simulink model "Lv_topo4"  (R2024a)
settings: Solver=ode4  StartTime=0.0  StopTime=1  FixedStep=5e-05  RelTol=1e-3
libraries: spsSeriesRLCBranchLib x38, spsThreePhaseSeriesRLCBranchLib x18, spsCurrentMeasurementLib x16, spsPowerLib x16, spsSeriesRLCLoadLib x16, spsVoltageMeasurementLib x16, spsThreePhaseVIMeasurementLib x2, spsGroundLib x2, spsPower3phInstantaneousLib x2, spsThreePhaseTransformerTwoWindingsLib x2, spsThreePhaseSourceLib x1, sps_lib x1
(part 2 of 2)

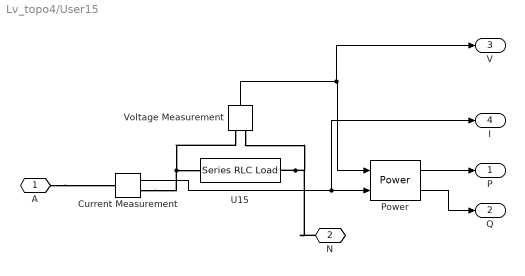
== system Lv_topo4/User15 ==
  Current Measurement : spsCurrentMeasurementLib/Current Measurement  PhasorSimulation=off  OutputType=Complex  PSBequivalent=0
  Power : spsPowerLib/Power  Freq=50  Vinit=[1, 0]  Iinit=[1, 0]  Ts=0
  U15 : spsSeriesRLCLoadLib/Series RLC Load  LConnTagsString=a  RConnTagsString=__new0  NominalVoltage=220  NominalFrequency=50  ActivePower=1045  InductivePower=503.5  CapacitivePower=0  Setx0=off  InitialVoltage=0  SetiL0=off  InitialCurrent=0  Measurements=None  LoadType=constant PQ
  Voltage Measurement : spsVoltageMeasurementLib/Voltage Measurement  PhasorSimulation=off  OutputType=Complex  PSBequivalent=0
  A : PMIOPort  Side=Left
  N : PMIOPort  Port=2  Side=Right
  P : Outport
  Q : Outport  Port=2
  V : Outport  Port=3
  I : Outport  Port=4
  wires:
  Power/1 -> P/1
  Power/2 -> Q/1
  Voltage Measurement/1 -> V/1, Power/1
  Current Measurement/1 -> I/1, Power/2
  connections:
  U15/RConn1 -- Voltage Measurement/LConn2 -- N/RConn1
  Current Measurement/RConn1 -- Voltage Measurement/LConn1 -- U15/LConn1
  A/RConn1 -- Current Measurement/LConn1

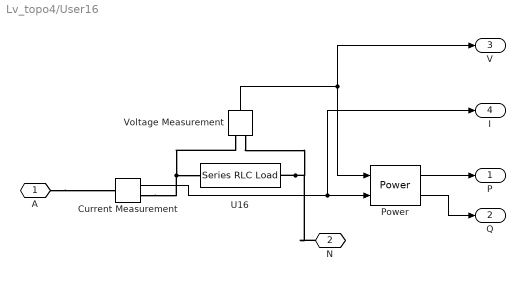
== system Lv_topo4/User16 ==
  Current Measurement : spsCurrentMeasurementLib/Current Measurement  PhasorSimulation=off  OutputType=Complex  PSBequivalent=0
  Power : spsPowerLib/Power  Freq=50  Vinit=[1, 0]  Iinit=[1, 0]  Ts=0
  U16 : spsSeriesRLCLoadLib/Series RLC Load  LConnTagsString=a  RConnTagsString=__new0  NominalVoltage=220  NominalFrequency=50  ActivePower=847  InductivePower=286  CapacitivePower=0  Setx0=off  InitialVoltage=0  SetiL0=off  InitialCurrent=0  Measurements=None  LoadType=constant PQ
  Voltage Measurement : spsVoltageMeasurementLib/Voltage Measurement  PhasorSimulation=off  OutputType=Complex  PSBequivalent=0
  A : PMIOPort  Side=Left
  N : PMIOPort  Port=2  Side=Right
  P : Outport
  Q : Outport  Port=2
  V : Outport  Port=3
  I : Outport  Port=4
  wires:
  Power/1 -> P/1
  Power/2 -> Q/1
  Current Measurement/1 -> I/1, Power/2
  Voltage Measurement/1 -> V/1, Power/1
  connections:
  U16/RConn1 -- Voltage Measurement/LConn2 -- N/RConn1
  Current Measurement/RConn1 -- Voltage Measurement/LConn1 -- U16/LConn1
  A/RConn1 -- Current Measurement/LConn1

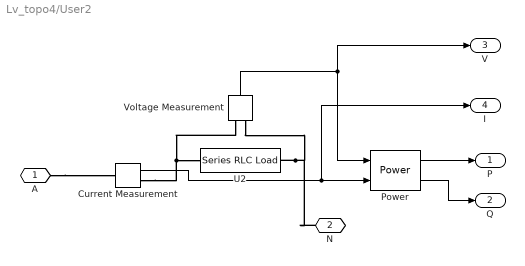
== system Lv_topo4/User2 ==
  Current Measurement : spsCurrentMeasurementLib/Current Measurement  PhasorSimulation=off  OutputType=Complex  PSBequivalent=0
  Power : spsPowerLib/Power  Freq=50  Vinit=[1, 0]  Iinit=[1, 0]  Ts=0
  U2 : spsSeriesRLCLoadLib/Series RLC Load  LConnTagsString=a  RConnTagsString=__new0  NominalVoltage=220  NominalFrequency=50  ActivePower=840  InductivePower=410  CapacitivePower=0  Setx0=off  InitialVoltage=0  SetiL0=off  InitialCurrent=0  Measurements=None  LoadType=constant PQ
  Voltage Measurement : spsVoltageMeasurementLib/Voltage Measurement  PhasorSimulation=off  OutputType=Complex  PSBequivalent=0
  A : PMIOPort  Side=Left
  N : PMIOPort  Port=2  Side=Right
  P : Outport
  Q : Outport  Port=2
  V : Outport  Port=3
  I : Outport  Port=4
  wires:
  Power/1 -> P/1
  Power/2 -> Q/1
  Voltage Measurement/1 -> V/1, Power/1
  Current Measurement/1 -> I/1, Power/2
  connections:
  U2/RConn1 -- Voltage Measurement/LConn2 -- N/RConn1
  Current Measurement/RConn1 -- Voltage Measurement/LConn1 -- U2/LConn1
  A/RConn1 -- Current Measurement/LConn1

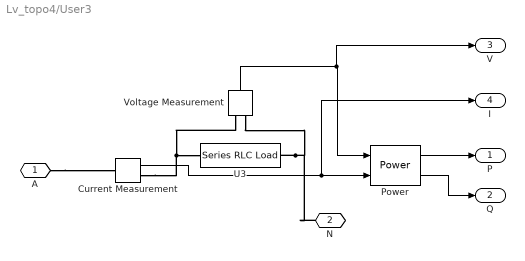
== system Lv_topo4/User3 ==
  Current Measurement : spsCurrentMeasurementLib/Current Measurement  PhasorSimulation=off  OutputType=Complex  PSBequivalent=0
  Power : spsPowerLib/Power  Freq=50  Vinit=[1, 0]  Iinit=[1, 0]  Ts=0
  U3 : spsSeriesRLCLoadLib/Series RLC Load  LConnTagsString=a  RConnTagsString=__new0  NominalVoltage=220  NominalFrequency=50  ActivePower=729.6  InductivePower=355.2  CapacitivePower=0  Setx0=off  InitialVoltage=0  SetiL0=off  InitialCurrent=0  Measurements=None  LoadType=constant PQ
  Voltage Measurement : spsVoltageMeasurementLib/Voltage Measurement  PhasorSimulation=off  OutputType=Complex  PSBequivalent=0
  A : PMIOPort  Side=Left
  N : PMIOPort  Port=2  Side=Right
  P : Outport
  Q : Outport  Port=2
  V : Outport  Port=3
  I : Outport  Port=4
  wires:
  Power/1 -> P/1
  Power/2 -> Q/1
  Current Measurement/1 -> I/1, Power/2
  Voltage Measurement/1 -> V/1, Power/1
  connections:
  U3/RConn1 -- Voltage Measurement/LConn2 -- N/RConn1
  Current Measurement/RConn1 -- Voltage Measurement/LConn1 -- U3/LConn1
  A/RConn1 -- Current Measurement/LConn1

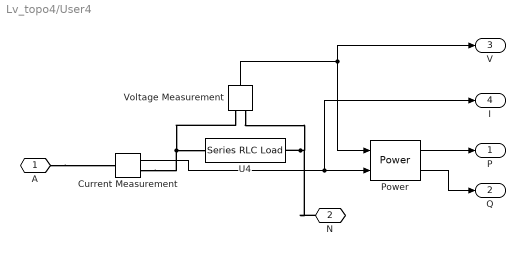
== system Lv_topo4/User4 ==
  Current Measurement : spsCurrentMeasurementLib/Current Measurement  PhasorSimulation=off  OutputType=Complex  PSBequivalent=0
  Power : spsPowerLib/Power  Freq=50  Vinit=[1, 0]  Iinit=[1, 0]  Ts=0
  U4 : spsSeriesRLCLoadLib/Series RLC Load  LConnTagsString=a  RConnTagsString=__new0  NominalVoltage=220  NominalFrequency=50  ActivePower=720  InductivePower=351  CapacitivePower=0  Setx0=off  InitialVoltage=0  SetiL0=off  InitialCurrent=0  Measurements=None  LoadType=constant PQ
  Voltage Measurement : spsVoltageMeasurementLib/Voltage Measurement  PhasorSimulation=off  OutputType=Complex  PSBequivalent=0
  A : PMIOPort  Side=Left
  N : PMIOPort  Port=2  Side=Right
  P : Outport
  Q : Outport  Port=2
  V : Outport  Port=3
  I : Outport  Port=4
  wires:
  Power/1 -> P/1
  Power/2 -> Q/1
  Voltage Measurement/1 -> V/1, Power/1
  Current Measurement/1 -> I/1, Power/2
  connections:
  U4/RConn1 -- Voltage Measurement/LConn2 -- N/RConn1
  Current Measurement/RConn1 -- Voltage Measurement/LConn1 -- U4/LConn1
  A/RConn1 -- Current Measurement/LConn1

== system Lv_topo4/User5 ==
  Current Measurement : spsCurrentMeasurementLib/Current Measurement  PhasorSimulation=off  OutputType=Complex  PSBequivalent=0
  Power : spsPowerLib/Power  Freq=50  Vinit=[1, 0]  Iinit=[1, 0]  Ts=0
  U5 : spsSeriesRLCLoadLib/Series RLC Load  LConnTagsString=a  RConnTagsString=__new0  NominalVoltage=220  NominalFrequency=50  ActivePower=1317.5  InductivePower=641.75  CapacitivePower=0  Setx0=off  InitialVoltage=0  SetiL0=off  InitialCurrent=0  Measurements=None  LoadType=constant PQ
  Voltage Measurement : spsVoltageMeasurementLib/Voltage Measurement  PhasorSimulation=off  OutputType=Complex  PSBequivalent=0
  A : PMIOPort  Side=Left
  N : PMIOPort  Port=2  Side=Right
  P : Outport
  Q : Outport  Port=2
  V : Outport  Port=3
  I : Outport  Port=4
  wires:
  Power/1 -> P/1
  Power/2 -> Q/1
  Current Measurement/1 -> I/1, Power/2
  Voltage Measurement/1 -> V/1, Power/1
  connections:
  U5/RConn1 -- Voltage Measurement/LConn2 -- N/RConn1
  Current Measurement/RConn1 -- Voltage Measurement/LConn1 -- U5/LConn1
  A/RConn1 -- Current Measurement/LConn1

== system Lv_topo4/User6 ==
  Current Measurement : spsCurrentMeasurementLib/Current Measurement  PhasorSimulation=off  OutputType=Complex  PSBequivalent=0
  Power : spsPowerLib/Power  Freq=50  Vinit=[1, 0]  Iinit=[1, 0]  Ts=0
  U6 : spsSeriesRLCLoadLib/Series RLC Load  LConnTagsString=a  RConnTagsString=__new0  NominalVoltage=220  NominalFrequency=50  ActivePower=1071  InductivePower=518.5  CapacitivePower=0  Setx0=off  InitialVoltage=0  SetiL0=off  InitialCurrent=0  Measurements=None  LoadType=constant PQ
  Voltage Measurement : spsVoltageMeasurementLib/Voltage Measurement  PhasorSimulation=off  OutputType=Complex  PSBequivalent=0
  A : PMIOPort  Side=Left
  N : PMIOPort  Port=2  Side=Right
  P : Outport
  Q : Outport  Port=2
  V : Outport  Port=3
  I : Outport  Port=4
  wires:
  Power/1 -> P/1
  Power/2 -> Q/1
  Voltage Measurement/1 -> V/1, Power/1
  Current Measurement/1 -> I/1, Power/2
  connections:
  U6/RConn1 -- Voltage Measurement/LConn2 -- N/RConn1
  Current Measurement/RConn1 -- Voltage Measurement/LConn1 -- U6/LConn1
  A/RConn1 -- Current Measurement/LConn1

== system Lv_topo4/User7 ==
  Current Measurement : spsCurrentMeasurementLib/Current Measurement  PhasorSimulation=off  OutputType=Complex  PSBequivalent=0
  Power : spsPowerLib/Power  Freq=50  Vinit=[1, 0]  Iinit=[1, 0]  Ts=0
  U7 : spsSeriesRLCLoadLib/Series RLC Load  LConnTagsString=a  RConnTagsString=__new0  NominalVoltage=220  NominalFrequency=50  ActivePower=570  InductivePower=275  CapacitivePower=0  Setx0=off  InitialVoltage=0  SetiL0=off  InitialCurrent=0  Measurements=None  LoadType=constant PQ
  Voltage Measurement : spsVoltageMeasurementLib/Voltage Measurement  PhasorSimulation=off  OutputType=Complex  PSBequivalent=0
  A : PMIOPort  Side=Left
  N : PMIOPort  Port=2  Side=Right
  P : Outport
  Q : Outport  Port=2
  V : Outport  Port=3
  I : Outport  Port=4
  wires:
  Power/1 -> P/1
  Power/2 -> Q/1
  Current Measurement/1 -> I/1, Power/2
  Voltage Measurement/1 -> V/1, Power/1
  connections:
  U7/RConn1 -- Voltage Measurement/LConn2 -- N/RConn1
  Current Measurement/RConn1 -- Voltage Measurement/LConn1 -- U7/LConn1
  A/RConn1 -- Current Measurement/LConn1

== system Lv_topo4/User8 ==
  Current Measurement : spsCurrentMeasurementLib/Current Measurement  PhasorSimulation=off  OutputType=Complex  PSBequivalent=0
  Power : spsPowerLib/Power  Freq=50  Vinit=[1, 0]  Iinit=[1, 0]  Ts=0
  U8 : spsSeriesRLCLoadLib/Series RLC Load  LConnTagsString=a  RConnTagsString=__new0  NominalVoltage=220  NominalFrequency=50  ActivePower=1080  InductivePower=522  CapacitivePower=0  Setx0=off  InitialVoltage=0  SetiL0=off  InitialCurrent=0  Measurements=None  LoadType=constant PQ
  Voltage Measurement : spsVoltageMeasurementLib/Voltage Measurement  PhasorSimulation=off  OutputType=Complex  PSBequivalent=0
  A : PMIOPort  Side=Left
  N : PMIOPort  Port=2  Side=Right
  P : Outport
  Q : Outport  Port=2
  V : Outport  Port=3
  I : Outport  Port=4
  wires:
  Power/1 -> P/1
  Power/2 -> Q/1
  Current Measurement/1 -> I/1, Power/2
  Voltage Measurement/1 -> V/1, Power/1
  connections:
  U8/RConn1 -- Voltage Measurement/LConn2 -- N/RConn1
  Current Measurement/RConn1 -- Voltage Measurement/LConn1 -- U8/LConn1
  A/RConn1 -- Current Measurement/LConn1

== system Lv_topo4/User9 ==
  Current Measurement : spsCurrentMeasurementLib/Current Measurement  PhasorSimulation=off  OutputType=Complex  PSBequivalent=0
  Power : spsPowerLib/Power  Freq=50  Vinit=[1, 0]  Iinit=[1, 0]  Ts=0
  U9 : spsSeriesRLCLoadLib/Series RLC Load  LConnTagsString=a  RConnTagsString=__new0  NominalVoltage=220  NominalFrequency=50  ActivePower=1530  InductivePower=918  CapacitivePower=0  Setx0=off  InitialVoltage=0  SetiL0=off  InitialCurrent=0  Measurements=None  LoadType=constant PQ
  Voltage Measurement : spsVoltageMeasurementLib/Voltage Measurement  PhasorSimulation=off  OutputType=Complex  PSBequivalent=0
  A : PMIOPort  Side=Left
  N : PMIOPort  Port=2  Side=Right
  P : Outport
  Q : Outport  Port=2
  V : Outport  Port=3
  I : Outport  Port=4
  wires:
  Power/1 -> P/1
  Power/2 -> Q/1
  Voltage Measurement/1 -> V/1, Power/1
  Current Measurement/1 -> I/1, Power/2
  connections:
  Voltage Measurement/LConn2 -- N/RConn1 -- U9/RConn1
  Voltage Measurement/LConn1 -- U9/LConn1 -- Current Measurement/RConn1
  A/RConn1 -- Current Measurement/LConn1
